simulink subsystem "Circuit_Under_Test"  (R2024b)
settings: Solver=VariableStepAuto  StartTime=0.0  StopTime=10.0  RelTol=1e-3
undefined symbols (not defined in the file or in its folder): Batt
libraries: fl_lib x6
settings Model: Creator=JesseJabezArendse  LastModifiedBy=JesseJabezArendse

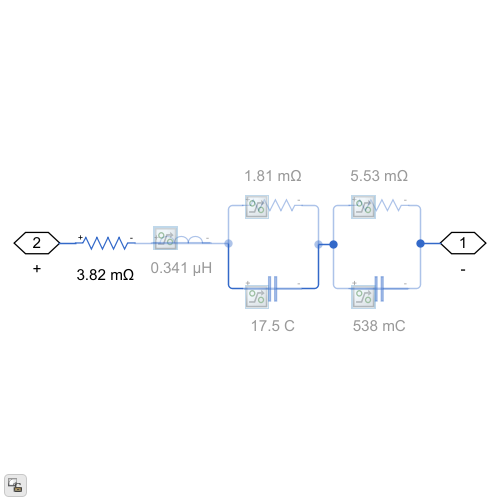
[thumbnail: Simulink's stored preview of the top-level diagram]
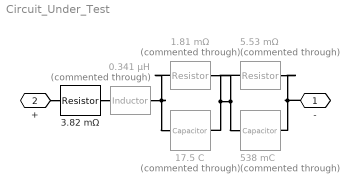
== system Circuit_Under_Test ==
  0.341 µH : fl_lib/Electrical/Electrical Elements/Inductor  Commented=through  l=Batt.L_R H  r=0 Ohm  g=0 1/Ohm  i_specify=off  i_priority=None  i=0 A  i_nominal_specify=off  i_nominal_value=1  i_nominal_unit=A  v_specify=off  v_priority=None  v=0 V  v_nominal_specify=off  v_nominal_value=1  v_nominal_unit=V  i_L_specify=off  i_L_priority=High  i_L=0 A  i_L_nominal_specify=off  i_L_nominal_value=1  i_L_nominal_unit=A
  1.81 mΩ : fl_lib/Electrical/Electrical Elements/Resistor  Commented=through  R=Batt.R_1 Ohm  i_specify=off  i_priority=None  i=0 A  i_nominal_specify=off  i_nominal_value=1  i_nominal_unit=A  v_specify=off  v_priority=None  v=0 V  v_nominal_specify=off  v_nominal_value=1  v_nominal_unit=V
  17.5 C : fl_lib/Electrical/Electrical Elements/Capacitor  Commented=through  c=Batt.C_1 F  r=0 Ohm  g=0 1/Ohm  i_specify=off  i_priority=None  i=0 A  i_nominal_specify=off  i_nominal_value=1  i_nominal_unit=A  v_specify=off  v_priority=None  v=0 V  v_nominal_specify=off  v_nominal_value=1  v_nominal_unit=V  vc_specify=off  vc_priority=High  vc=0 V  vc_nominal_specify=off  vc_nominal_value=1  vc_nominal_unit=V
  3.82 mΩ : fl_lib/Electrical/Electrical Elements/Resistor  R=0.1 Ohm  i_specify=off  i_priority=None  i=0 A  i_nominal_specify=off  i_nominal_value=1  i_nominal_unit=A  v_specify=off  v_priority=None  v=0 V  v_nominal_specify=off  v_nominal_value=1  v_nominal_unit=V
  5.53 mΩ : fl_lib/Electrical/Electrical Elements/Resistor  Commented=through  R=Batt.R_2 Ohm  i_specify=off  i_priority=None  i=0 A  i_nominal_specify=off  i_nominal_value=1  i_nominal_unit=A  v_specify=off  v_priority=None  v=0 V  v_nominal_specify=off  v_nominal_value=1  v_nominal_unit=V
  538 mC : fl_lib/Electrical/Electrical Elements/Capacitor  Commented=through  c=Batt.C_2 F  r=0 Ohm  g=0 1/Ohm  i_specify=off  i_priority=None  i=0 A  i_nominal_specify=off  i_nominal_value=1  i_nominal_unit=A  v_specify=off  v_priority=None  v=0 V  v_nominal_specify=off  v_nominal_value=1  v_nominal_unit=V  vc_specify=off  vc_priority=High  vc=0 V  vc_nominal_specify=off  vc_nominal_value=1  vc_nominal_unit=V
  - : PMIOPort  Side=Right
  + : PMIOPort  Port=2  Side=Left
  connections:
  1.81 mΩ/RConn1 -- 17.5 C/RConn1 -- 5.53 mΩ/LConn1 -- 538 mC/LConn1
  -/RConn1 -- 538 mC/RConn1 -- 5.53 mΩ/RConn1
  0.341 µH/RConn1 -- 17.5 C/LConn1 -- 1.81 mΩ/LConn1
  3.82 mΩ/RConn1 -- 0.341 µH/LConn1
  +/RConn1 -- 3.82 mΩ/LConn1
